simulink model "MySimModel"  (R2024b)
settings: Solver=VariableStepAuto  StartTime=0.0  StopTime=10.0  RelTol=1e-3
libraries: fl_lib x6, nesl_utility x3
settings Model: Creator=xinxing  LastModifiedBy=xinxing

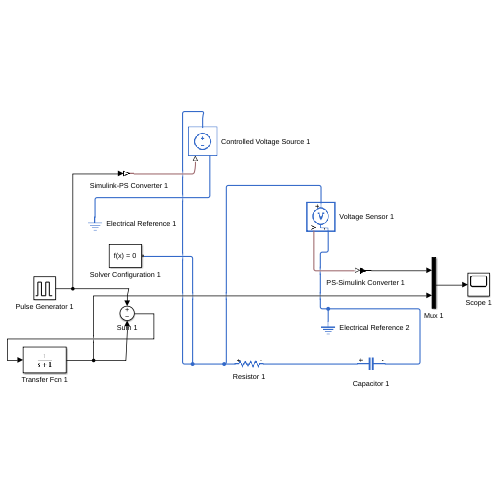
[thumbnail: Simulink's stored preview of the top-level diagram]
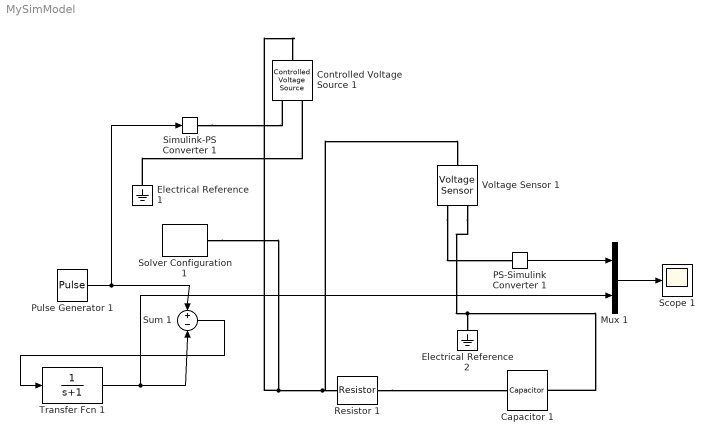
== system MySimModel ==
  Capacitor 1 : fl_lib/Electrical/Electrical Elements/Capacitor  c=1e-6 F  r=1e-6 Ohm  g=0 1/Ohm  i_specify=off  i_priority=None  i=0 A  i_nominal_specify=off  i_nominal_value=1  i_nominal_unit=A  v_specify=off  v_priority=None  v=0 V  v_nominal_specify=off  v_nominal_value=1  v_nominal_unit=V  vc_specify=off  vc_priority=High  vc=0 V  vc_nominal_specify=off  vc_nominal_value=1  vc_nominal_unit=V
  Controlled Voltage Source 1 : fl_lib/Electrical/Electrical Sources/Controlled Voltage Source
  Electrical Reference 1 : fl_lib/Electrical/Electrical Elements/Electrical Reference
  Electrical Reference 2 : fl_lib/Electrical/Electrical Elements/Electrical Reference
  Mux 1 : Mux  Inputs=2
  PS-Simulink Converter 1 : nesl_utility/PS-Simulink Converter  PhysicalDomain=network_engine_domain  SubClassName=ps_output  LeftPortType=input  RightPortType=output  PseudoPeriodic=off  Frequencies=[]  VectorFormat=inherit  Unit=inherit  AffineConversion=off
  Pulse Generator 1 : DiscretePulseGenerator  PulseType=Time based  Period=10  PulseWidth=5
  Resistor 1 : fl_lib/Electrical/Electrical Elements/Resistor  R=1 Ohm  i_specify=off  i_priority=None  i=0 A  i_nominal_specify=off  i_nominal_value=1  i_nominal_unit=A  v_specify=off  v_priority=None  v=0 V  v_nominal_specify=off  v_nominal_value=1  v_nominal_unit=V
  Scope 1 : Scope
  Simulink-PS Converter 1 : nesl_utility/Simulink-PS Converter  PhysicalDomain=network_engine_domain  SubClassName=ps_input  LeftPortType=input  RightPortType=output  PseudoPeriodic=off  Frequencies=[]  NoiseDistribution=none  NoiseParameters=[]  Unit=1  AffineConversion=off  FilteringAndDerivatives=provide  SimscapeFilterOrder=1  InputFilterTimeConstant=0.001  UdotUserProvided=0
  Solver Configuration 1 : nesl_utility/Solver Configuration  PhysicalDomain=network_engine_domain  SubClassName=solver  LeftPortType=input  RightPortType=generic  Tones=[]  Harmonics=[]  SimulateNoise=off  Profile=off  UseLocalSampling=off  EnableSwitchedLinearOptims=on  FrequencyDomain=off  UseCCode=off  RelTol=0.001  AbsTol=0.001  MinStep=1e-09  ToWorkspace=off  RevertToSquareIcSolve=off  NumHomotopyIterations=100  PhasorMode=off  PhasorModeNumHarmonics=1  ConsistencySolver=NEWTON_XTOL_AFTER_FTOL  IndexReductionMethod=DerivativeReplacement  DoDC=off  ResidualTolerance=1e-09  ConsistencyTolSource=GLOBAL  ConsistencyAbsTol=0.001  ConsistencyRelTol=0.001  ConsistencyTolFactor=0.001  UseLocalSolver=off  LocalSolverChoice=NE_BACKWARD_EULER_ADVANCER  ResolveIndetEquations=on  FunctionEvalNumThread=1  LocalSolverSampleTime=0.001  DoFixedCost=off  MaxNonlinIter=3  MaxModeIter=2  ComputeImpulses=off  ImpulseIterations=2  LinearAlgebra=auto  LinearAlgebraNumThread=0  EquationFormulation=NE_TIME_EF  DelaysMemoryBudget=1024  AutomaticFiltering=on  FilteringTimeConstant=0.001  PartitionStorageMethod=AS_NEEDED  PartitionMemoryBudget=1024  PartitionMethod=ROBUST  MultibodyUseLocalSolver=off  MultibodyLocalSolverChoice=ODE1  MultibodyLocalSolverSampleTime=0.001
  Sum 1 : Sum  Inputs=+-
  Transfer Fcn 1 : TransferFcn  Denominator=[1 1]
  Voltage Sensor 1 : fl_lib/Electrical/Electrical Sensors/Voltage Sensor
  wires:
  Mux 1/1 -> Scope 1/1
  PS-Simulink Converter 1/1 -> Mux 1/1
  Sum 1/1 -> Transfer Fcn 1/1
  Transfer Fcn 1/1 -> Sum 1/2, Mux 1/2
  Pulse Generator 1/1 -> Simulink-PS Converter 1/1, Sum 1/1
  connections:
  Resistor 1/RConn1 -- Capacitor 1/LConn1
  Voltage Sensor 1/RConn2 -- Electrical Reference 2/LConn1 -- Capacitor 1/RConn1
  Solver Configuration 1/RConn1 -- Resistor 1/LConn1 -- Voltage Sensor 1/LConn1 -- Controlled Voltage Source 1/LConn1
  Electrical Reference 1/LConn1 -- Controlled Voltage Source 1/RConn2
  Voltage Sensor 1/RConn1 -- PS-Simulink Converter 1/LConn1
  Simulink-PS Converter 1/RConn1 -- Controlled Voltage Source 1/RConn1
